simulink model "F16_DS3_ALTITUDE_SIMULINK"  (R2021b)
settings: Solver=VariableStepAuto  StartTime=0.0  StopTime=100  RelTol=1e-3
model workspace (MAT data in the model file):
  simin = 80
undefined symbols (not defined in the file or in its folder): input
settings Model: PacingRate=100  Creator=MARCELO  LastModifiedBy=MARCELO

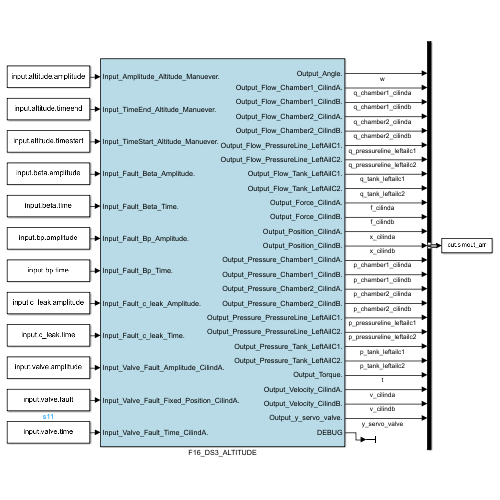
[thumbnail: Simulink's stored preview of the top-level diagram]
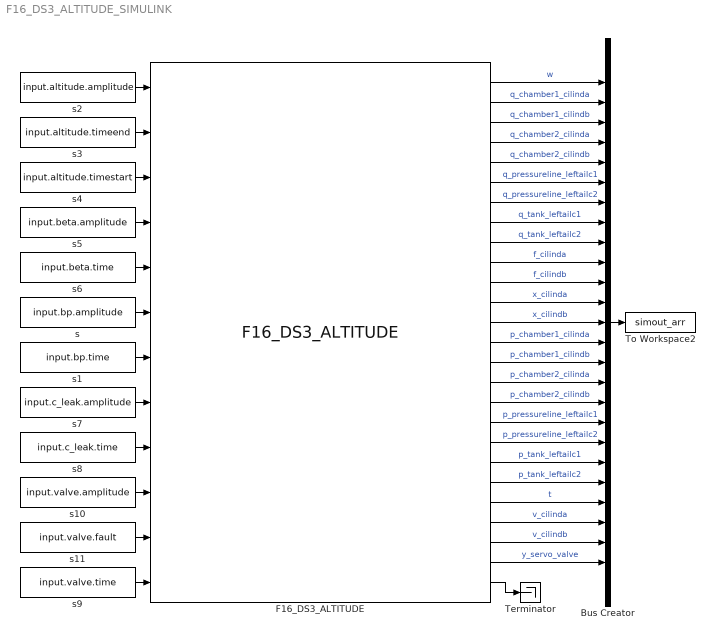
== system F16_DS3_ALTITUDE_SIMULINK ==
  Bus Creator : BusCreator  Inputs=25
  F16_DS3_ALTITUDE : S-Function  FunctionName=F16_DS3_ALTITUDE  SFunctionDeploymentMode=off  EnableBusSupport=off
      mask Display: port_label('input',1,'Input_Amplitude_Altitude_Manuever.'); port_label('input',2,'Input_TimeEnd_Altitude_Manuever.'); port_label('input',3,'Input_TimeStart_Altitude_Manuever.'); port_label('input',4,'Input_Fault_Beta_Amplitude.'); port_label('input',5,'Input_Fault_Beta_Time.'); port_label('input',6,'Input_Fault_Bp_Amplitude.'); port_label('input',7,'Input_Fault_Bp_Time.'); port_label('input',8,'Input_Fault_c_leak_Amplitude.'); port_label('input',9,'Input_Fault_c_leak_Time.'); port_label('input',10,'Input_Valve_Fault_Amplitude_CilindA.'); port_label('input',11,'Input_Valve_Fault_Fixed_Position_CilindA.'); port_label('input',12,'Input_Valve_Fault_Time_CilindA.'); port_label('output',1,'Output_Angle.'); port_label('output',2,'Output_Flow_Chamber1_CilindA.'); port_label('output',3,'Output_Flow_Chamber1_CilindB.'); port_label('output',4,'Output_Flow_Chamber2_CilindA.'); port_label('output',5,'Output_Flow_Chamber2_CilindB.'); port_label('output',6,'Output_Flow_PressureLine_LeftAilC1.'); port_label('output',7,'Output_Flow_PressureLine_LeftAilC2.'); port_label('output',8,'Output_Flow_Tank_LeftAilC1.'); port_label('output',9,'Output_Flow_Tank_LeftAilC2.'); port_label('output',10,'Output_Force_CilindA.'); port_label('output',11,'Output_Force_CilindB.'); port_label('output',12,'Output_Position_CilindA.'); port_label('output',13,'Output_Position_CilindB.'); port_label('output',14,'Output_Pressure_Chamber1_CilindA.'); port_label('output',15,'Output_Pressure_Chamber1_CilindB.'); port_label('output',16,'Output_Pressure_Chamber2_CilindA.'); port_label('output',17,'Output_Pressure_Chamber2_CilindB.'); port_label('output',18,'Output_Pressure_PressureLine_LeftAilC1.'); port_label('output',19,'Output_Pressure_PressureLine_LeftAilC2.'); port_label('output',20,'Output_Pressure_Tank_LeftAilC1.'); port_label('output',21,'Output_Pressure_Tank_LeftAilC2.'); port_label('output',22,'Output_Torque.'); port_label('output',23,'Output_Velocity_CilindA.'); port_label('output',24,'Output_Velocity_CilindB.'); port_label('output',25,'Output_y_servo_valve.'); port_label('output',26,'DEBUG')
  Terminator : Terminator
  To Workspace2 : ToWorkspace  VariableName=simout_arr  SampleTime=0.1
  s : Constant  Value=input.bp.amplitude
  s1 : Constant  Value=input.bp.time
  s10 : Constant  Value=input.valve.amplitude
  s11 : Constant  Value=input.valve.fault
  s2 : Constant  Value=input.altitude.amplitude
  s3 : Constant  Value=input.altitude.timeend
  s4 : Constant  Value=input.altitude.timestart
  s5 : Constant  Value=input.beta.amplitude
  s6 : Constant  Value=input.beta.time
  s7 : Constant  Value=input.c_leak.amplitude
  s8 : Constant  Value=input.c_leak.time
  s9 : Constant  Value=input.valve.time
  wires:
  s/1 -> F16_DS3_ALTITUDE/6
  s1/1 -> F16_DS3_ALTITUDE/7
  s9/1 -> F16_DS3_ALTITUDE/12
  s8/1 -> F16_DS3_ALTITUDE/9
  s7/1 -> F16_DS3_ALTITUDE/8
  s6/1 -> F16_DS3_ALTITUDE/5
  s5/1 -> F16_DS3_ALTITUDE/4
  s4/1 -> F16_DS3_ALTITUDE/3
  s3/1 -> F16_DS3_ALTITUDE/2
  s2/1 -> F16_DS3_ALTITUDE/1
  s10/1 -> F16_DS3_ALTITUDE/10
  s11/1 -> F16_DS3_ALTITUDE/11
  Bus Creator/1 -> To Workspace2/1
  F16_DS3_ALTITUDE/1 -> Bus Creator/1  "w"
  F16_DS3_ALTITUDE/2 -> Bus Creator/2  "q_chamber1_cilinda"
  F16_DS3_ALTITUDE/3 -> Bus Creator/3  "q_chamber1_cilindb"
  F16_DS3_ALTITUDE/4 -> Bus Creator/4  "q_chamber2_cilinda"
  F16_DS3_ALTITUDE/5 -> Bus Creator/5  "q_chamber2_cilindb"
  F16_DS3_ALTITUDE/6 -> Bus Creator/6  "q_pressureline_leftailc1"
  F16_DS3_ALTITUDE/7 -> Bus Creator/7  "q_pressureline_leftailc2"
  F16_DS3_ALTITUDE/8 -> Bus Creator/8  "q_tank_leftailc1"
  F16_DS3_ALTITUDE/9 -> Bus Creator/9  "q_tank_leftailc2"
  F16_DS3_ALTITUDE/10 -> Bus Creator/10  "f_cilinda"
  F16_DS3_ALTITUDE/11 -> Bus Creator/11  "f_cilindb"
  F16_DS3_ALTITUDE/12 -> Bus Creator/12  "x_cilinda"
  F16_DS3_ALTITUDE/13 -> Bus Creator/13  "x_cilindb"
  F16_DS3_ALTITUDE/14 -> Bus Creator/14  "p_chamber1_cilinda"
  F16_DS3_ALTITUDE/15 -> Bus Creator/15  "p_chamber1_cilindb"
  F16_DS3_ALTITUDE/16 -> Bus Creator/16  "p_chamber2_cilinda"
  F16_DS3_ALTITUDE/17 -> Bus Creator/17  "p_chamber2_cilindb"
  F16_DS3_ALTITUDE/18 -> Bus Creator/18  "p_pressureline_leftailc1"
  F16_DS3_ALTITUDE/19 -> Bus Creator/19  "p_pressureline_leftailc2"
  F16_DS3_ALTITUDE/20 -> Bus Creator/20  "p_tank_leftailc1"
  F16_DS3_ALTITUDE/21 -> Bus Creator/21  "p_tank_leftailc2"
  F16_DS3_ALTITUDE/22 -> Bus Creator/22  "t"
  F16_DS3_ALTITUDE/23 -> Bus Creator/23  "v_cilinda"
  F16_DS3_ALTITUDE/24 -> Bus Creator/24  "v_cilindb"
  F16_DS3_ALTITUDE/25 -> Bus Creator/25  "y_servo_valve"
  F16_DS3_ALTITUDE/26 -> Terminator/1
